simulink model "rst_auto_reg_complete_4a_2018b"  (R2018b)
settings: Solver=FixedStepAuto  StartTime=0.0  StopTime=200  RelTol=1e-3
values from neighbouring files (symbols this model uses):
  A = dend    [RST_2ordem_final.m]    (also in RST_4ordem_final.m)
  B = numd    [RST_2ordem_final.m]    (also in RST_4ordem_final.m)
  ep = 0.7    [RST_2ordem_final.m]    (also in RST_4ordem_final.m)
  initial_theta = [-0.31 -0.55 0.0021 0.12]    [RST_2ordem_final.m]    (also in RST_4ordem_final.m = [-1.0 0.38 0.07 0.23 0.03 0.12 0.06 0.005])
  Ta = 0.1    [RST_2ordem_final.m]    (also in RST_4ordem_final.m = 1)
  Tas = Ta    (= 0.1)    [RST_2ordem_final.m]    (also in RST_4ordem_final.m = 1)
  theta_switch_time = 10*Ta    (= 1)    [RST_2ordem_final.m]    (also in RST_4ordem_final.m = 10)
  Ts = 1    [RST_2ordem_final.m]    (also in RST_4ordem_final.m = 5)
  w0 = 1    [RST_2ordem_final.m]    (also in RST_4ordem_final.m = 0.1)
undefined symbols (not defined in the file or in its folder): R, S, T
libraries: dspinverses x6, simulink x2
(part 2 of 2)

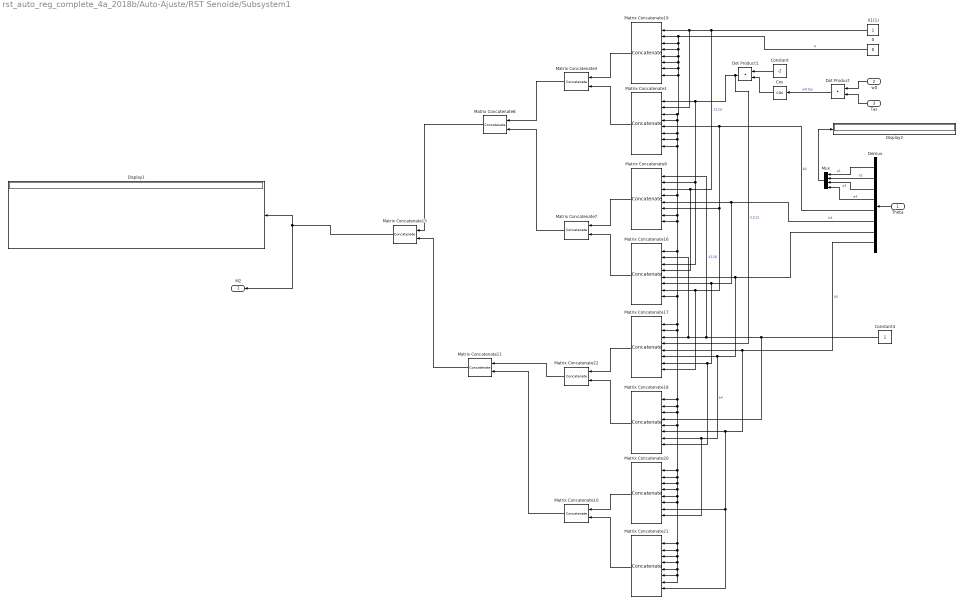
== system rst_auto_reg_complete_4a_2018b/Auto-Ajuste/RST Senoide/Subsystem1 ==
  Theta : Inport
  w0 : Inport  Port=2
  Tas : Inport  Port=3
  0 : Constant  Value=0
  Constant : Constant  Value=-2
  Constant4 : Constant
  Cos : Trigonometry  Operator=cos
  Demux : Demux  Outputs=8
  Display1 : Display
  Display3 : Display
  Dot Product : DotProduct  InputSameDT=on  OutDataTypeStr=Inherit: Inherit via internal rule
  Dot Product1 : DotProduct  InputSameDT=on  OutDataTypeStr=Inherit: Inherit via internal rule
  Matrix Concatenate{1,9,16..21} (8 alike) : Concatenate  NumInputs=8  Mode=Multidimensional array  ConcatenateDimension=2
  Matrix Concatenate{3,7..8,10..11,15,22} (7 alike) : Concatenate  Mode=Multidimensional array
  Mux : Mux
  X1(1) : Constant
  M2 : Outport
  wires:
  Matrix Concatenate1/1 -> Matrix Concatenate3/2
  Matrix Concatenate20/1 -> Matrix Concatenate10/1
  Matrix Concatenate21/1 -> Matrix Concatenate10/2
  Matrix Concatenate10/1 -> Matrix Concatenate11/2
  Matrix Concatenate11/1 -> Matrix Concatenate15/2
  Matrix Concatenate22/1 -> Matrix Concatenate11/1
  Matrix Concatenate18/1 -> Matrix Concatenate22/2
  Matrix Concatenate9/1 -> Matrix Concatenate7/1
  Matrix Concatenate17/1 -> Matrix Concatenate22/1
  Matrix Concatenate8/1 -> Matrix Concatenate15/1
  Matrix Concatenate16/1 -> Matrix Concatenate7/2
  Theta/1 -> Demux/1
  Matrix Concatenate3/1 -> Matrix Concatenate8/1
  Matrix Concatenate7/1 -> Matrix Concatenate8/2
  Matrix Concatenate19/1 -> Matrix Concatenate3/1
  X1(1)/1 -> Matrix Concatenate16/4, Matrix Concatenate9/3, Matrix Concatenate1/2, Matrix Concatenate19/1  "X1(1)"
  Demux/1 -> Mux/1  "a1"
  Demux/2 -> Mux/2  "a2"
  Demux/3 -> Mux/3  "a3"
  Demux/4 -> Mux/4  "a4"
  Mux/1 -> Display3/1
  0/1 -> Matrix Concatenate19/5, Matrix Concatenate1/6, Matrix Concatenate9/7, Matrix Concatenate16/8, Matrix Concatenate18/5, Matrix Concatenate20/1, Matrix Concatenate20/4, Matrix Concatenate21/7, Matrix Concatenate21/6, Matrix Concatenate21/5, Matrix Concatenate21/4, Matrix Concatenate21/3, Matrix Concatenate21/2, Matrix Concatenate21/1, Matrix Concatenate20/6, Matrix Concatenate20/5, Matrix Concatenate20/3, Matrix Concatenate20/2, Matrix Concatenate18/3, Matrix Concatenate18/2, Matrix Concatenate18/1, Matrix Concatenate17/2, Matrix Concatenate17/1, Matrix Concatenate16/1, Matrix Concatenate9/8, Matrix Concatenate9/4, Matrix Concatenate1/8, Matrix Concatenate1/7, Matrix Concatenate1/4, Matrix Concatenate1/3, Matrix Concatenate19/8, Matrix Concatenate19/7, Matrix Concatenate19/6, Matrix Concatenate19/4, Matrix Concatenate19/3, Matrix Concatenate19/2  "0"
  Matrix Concatenate15/1 -> M2/1, Display1/1
  Demux/5 -> Matrix Concatenate17/8, Matrix Concatenate16/7, Matrix Concatenate9/6, Matrix Concatenate1/5  "b2"
  Demux/6 -> Matrix Concatenate18/8, Matrix Concatenate17/7, Matrix Concatenate16/6, Matrix Concatenate9/5  "b3"
  Demux/7 -> Matrix Concatenate20/8, Matrix Concatenate18/7, Matrix Concatenate17/6, Matrix Concatenate16/5  "b4"
  Demux/8 -> Matrix Concatenate21/8, Matrix Concatenate20/7, Matrix Concatenate18/6, Matrix Concatenate17/5  "b5"
  Constant/1 -> Dot Product1/1
  Cos/1 -> Dot Product1/2
  Tas/1 -> Dot Product/2
  w0/1 -> Dot Product/1
  Dot Product/1 -> Cos/1  "w0.tas"
  Dot Product1/1 -> Matrix Concatenate17/4, Matrix Concatenate16/3, Matrix Concatenate9/2, Matrix Concatenate1/1  "X1(2)"
  Constant4/1 -> Matrix Concatenate18/4, Matrix Concatenate9/1, Matrix Concatenate16/2, Matrix Concatenate17/3  "X1(3)"
